simulink model "control_parqueadero"  (R2020b)
settings: Solver=VariableStepAuto  StartTime=0.0  StopTime=inf  RelTol=1e-3
settings Model: Creator=mateo  LastModifiedBy=mateo
settings OptimizationCC: DefaultParameterBehavior=Inlined  UseDivisionForNetSlopeComputation=on  GainParamInheritBuiltInType=on  UseFloatMulNetSlope=on  InlineInvariantSignals=on  PassReuseOutputArgsAs=Individual arguments  ZeroExternalMemoryAtStartup=off  ZeroInternalMemoryAtStartup=off  NoFixptDivByZeroProtection=on  EfficientFloat2IntCast=on  LifeSpan=1  OptimizeBlockOrder=speed  DifferentSizesBufferReuse=on  EfficientTunableParamExpr=on
settings DebuggingCC: ParameterTunabilityLossMsg=error
settings HardwareCC: ProdLongLongMode=on
settings SFSimCC: MATLABDynamicMemAlloc=off
settings RTWCC: Description=Embedded Coder  SystemTargetFile=ert.tlc  TemplateMakefile=ert_default_tmf  GenerateReport=on  LaunchReport=on  GenerateWebview=on
settings CodeAppCC: ForceParamTrailComments=on  IgnoreCustomStorageClasses=off  OperatorAnnotations=on  SimulinkDataObjDesc=on  SFDataObjDesc=on  CustomSymbolStrGlobalVar=rt$N$M  CustomSymbolStrType=$N$M  CustomSymbolStrFcn=$N$M$F  CustomSymbolStrMacro=$N$M  InsertBlockDesc=on
settings ERTTargetCC: TargetLangStandard=C99 (ISO)  GenerateSampleERTMain=on  IncludeMdlTerminateFcn=off  CombineSignalStateStructs=on  SupportComplex=off  SupportContinuousTime=on  SupportNonInlinedSFcns=on  InlinedParameterPlacement=NonHierarchical  ERTCustomFileTemplate=example_file_process.tlc  ERTFilePackagingFormat=CompactWithDataFile

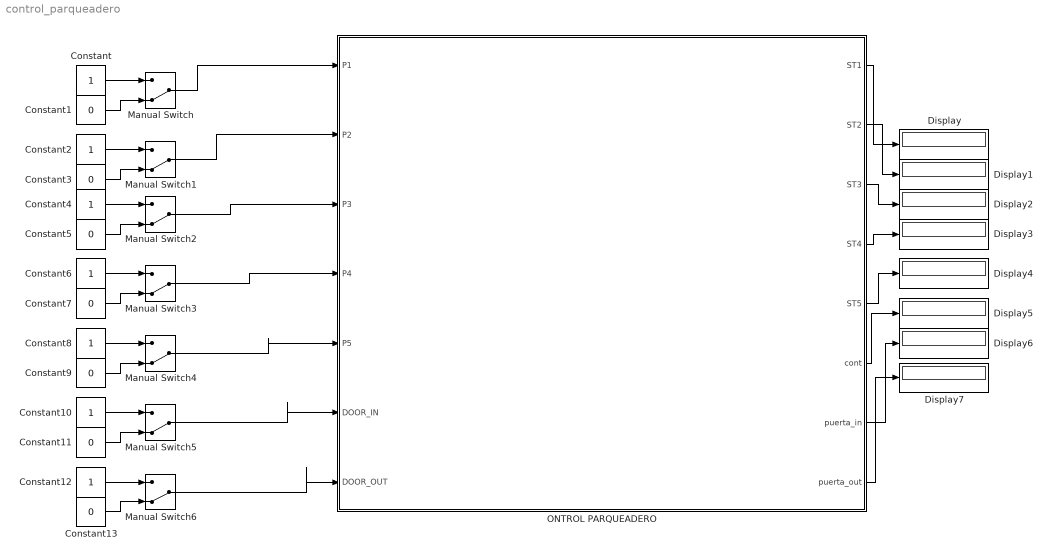
== system control_parqueadero ==
  Constant{,2,4,6,8,10,12} (7 alike) : Constant
  Constant{1,3,5,7,9,11,13} (7 alike) : Constant  Value=0
  Display{,1..7} (8 alike) : Display
  Manual Switch{,1..6} (7 alike) : ManualSwitch  CurrentSetting=0
  ONTROL PARQUEADERO : Subsystem
  wires:
  Constant/1 -> Manual Switch/1
  Constant1/1 -> Manual Switch/2
  Constant3/1 -> Manual Switch1/2
  Constant2/1 -> Manual Switch1/1
  Constant4/1 -> Manual Switch2/1
  Constant5/1 -> Manual Switch2/2
  Constant7/1 -> Manual Switch3/2
  Constant6/1 -> Manual Switch3/1
  Constant8/1 -> Manual Switch4/1
  Constant9/1 -> Manual Switch4/2
  Constant11/1 -> Manual Switch5/2
  Constant10/1 -> Manual Switch5/1
  Constant12/1 -> Manual Switch6/1
  Constant13/1 -> Manual Switch6/2
  Manual Switch/1 -> ONTROL PARQUEADERO/1(P1)
  Manual Switch1/1 -> ONTROL PARQUEADERO/2(P2)
  Manual Switch2/1 -> ONTROL PARQUEADERO/3(P3)
  Manual Switch3/1 -> ONTROL PARQUEADERO/4(P4)
  Manual Switch4/1 -> ONTROL PARQUEADERO/5(P5)
  Manual Switch5/1 -> ONTROL PARQUEADERO/6(DOOR_IN)
  Manual Switch6/1 -> ONTROL PARQUEADERO/7(DOOR_OUT)
  ONTROL PARQUEADERO/1(ST1) -> Display/1
  ONTROL PARQUEADERO/2(ST2) -> Display1/1
  ONTROL PARQUEADERO/3(ST3) -> Display2/1
  ONTROL PARQUEADERO/4(ST4) -> Display3/1
  ONTROL PARQUEADERO/5(ST5) -> Display4/1
  ONTROL PARQUEADERO/6(cont) -> Display5/1
  ONTROL PARQUEADERO/7(puerta_in) -> Display6/1
  ONTROL PARQUEADERO/8(puerta_out) -> Display7/1

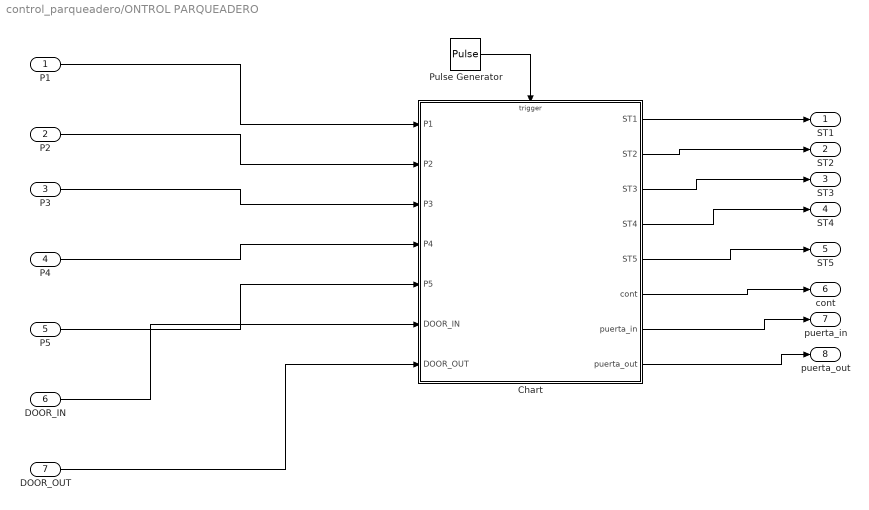
== system control_parqueadero/ONTROL PARQUEADERO ==
  P1 : Inport
  P2 : Inport  Port=2
  P3 : Inport  Port=3
  P4 : Inport  Port=4
  P5 : Inport  Port=5
  DOOR_IN : Inport  Port=6
  DOOR_OUT : Inport  Port=7
  Chart : Stateflow chart  TreatAsAtomicUnit=on
  Pulse Generator : DiscretePulseGenerator  PulseType=Time based  Period=1/1000  PulseWidth=50
  ST1 : Outport
  ST2 : Outport  Port=2
  ST3 : Outport  Port=3
  ST4 : Outport  Port=4
  ST5 : Outport  Port=5
  cont : Outport  Port=6
  puerta_in : Outport  Port=7
  puerta_out : Outport  Port=8
  wires:
  P4/1 -> Chart/4(P4)
  Chart/5(ST5) -> ST5/1
  P5/1 -> Chart/5(P5)
  Chart/2(ST2) -> ST2/1
  P1/1 -> Chart/1(P1)
  Pulse Generator/1 -> Chart/Trigger
  Chart/8(puerta_out) -> puerta_out/1
  DOOR_OUT/1 -> Chart/7(DOOR_OUT)
  DOOR_IN/1 -> Chart/6(DOOR_IN)
  Chart/7(puerta_in) -> puerta_in/1
  Chart/1(ST1) -> ST1/1
  Chart/3(ST3) -> ST3/1
  P2/1 -> Chart/2(P2)
  P3/1 -> Chart/3(P3)
  Chart/6(cont) -> cont/1
  Chart/4(ST4) -> ST4/1

== stateflow chart control_parqueadero/ONTROL PARQUEADERO/Chart ==
  state PARQ1_ON
    entry:
    ST1=1;
  state PARQ1_OFF
    entry:
    ST1=0;
  state PARQ2_ON
    entry:
    ST2=1;
  state PARQ2_OFF
    entry:
    ST2=0;
  state aumentar
    entry:
    puerta_in=0;
    cont1=cont1+1;
    cont=cont+1;
  state INICIO
    entry:
    ST1=0;
    ST2=0;
    ST3=0;
    ST4=0;
    ST5=0;
  state abrir
    entry:
    puerta_in=1
  state PARQ3_ON
    entry:
    ST3=1;
  state PARQ3_OFF
    entry:
    ST3=0;
  state abrir1
    entry:
    puerta_out=1
  state PARQ4_ON
    entry:
    ST4=1;
  state disminuir
    entry:
    puerta_out=0;
    cont1=cont1-1;
    cont=cont-1;
  state PARQ4_OFF
    entry:
    ST4=0;
  state PARQ5_ON
    entry:
    ST5=1;
  state PARQ5_OFF
    entry:
    ST5=0;
  (junction 72) -> abrir [order 2] : [DOOR_IN==1]
  (junction 72) -> abrir1 [order 3] : [DOOR_OUT==1]
  PARQ1_ON -> (junction 72)
  aumentar -> PARQ1_ON [order 1] : [P1==1]
  PARQ1_OFF -> (junction 91)
  disminuir -> PARQ1_OFF [order 1] : [P1==0]
  (junction 72) -> (junction 80) [order 1] : [cont1==5]
  PARQ2_ON -> (junction 72)
  (junction 91) -> (junction 72)
  (junction 80) -> abrir1 : [DOOR_OUT==1]
  PARQ3_ON -> (junction 72)
  PARQ5_ON -> (junction 72)
  PARQ4_ON -> (junction 72)
  aumentar -> PARQ2_ON [order 2] : [P2==1]
  disminuir -> PARQ2_OFF [order 2] : [P2==0]
  PARQ2_OFF -> (junction 91)
  (default) -> INICIO
  INICIO -> abrir [order 2] : [DOOR_IN==1]
  abrir -> aumentar : [DOOR_IN==0]
  aumentar -> PARQ3_ON [order 3] : [P3==1]
  aumentar -> PARQ5_ON [order 5] : [P5==1]
  aumentar -> PARQ4_ON [order 4] : [P4==1]
  INICIO -> abrir1 [order 1] : [DOOR_OUT==1]
  PARQ3_OFF -> (junction 91)
  disminuir -> PARQ3_OFF [order 3] : [P3==0]
  PARQ4_OFF -> (junction 91)
  PARQ5_OFF -> (junction 91)
  abrir1 -> disminuir : [DOOR_OUT==0]
  disminuir -> PARQ4_OFF [order 4] : [P4==0]
  disminuir -> PARQ5_OFF [order 5] : [P5==0]
  data: P1 input; P2 input; P3 input; P4 input; P5 input; ST1 output =0; ST2 output =0; ST3 output =0; ST4 output =0; ST5 output =0; DOOR_IN input; DOOR_OUT input; cont output =0; cont1 local =0; puerta_in output =0; puerta_out output =0
  events: clock input EITHER_EDGE_EVENT
